simulink model "DSC_filtering"  (R2022a)
settings: Solver=FixedStepDiscrete  StartTime=0.0  StopTime=Inf  FixedStep=100e-6  RelTol=1e-3  EnableMultiTasking=on
undefined symbols (not defined in the file): Num
settings Model: ExtModeEnableFloating=off  ExtModeTrigType=signal  ExtModeTrigDuration=1001  ExtModeTrigLevel=0.500000  ExtModeArchiveMode=auto  ExtModeArchiveFileName=Simulation  ExtModeArchiveDirName=C:\Users\05983057\Documents\MATLAB\practica2\03_DSC  ExtModeLogAll=off  Creator=05983057  LastModifiedBy=05983057
settings DataIOCC: ReturnWorkspaceOutputs=off
settings OptimizationCC: DefaultUnderspecifiedDataType=single  EnhancedBackFolding=on  PassReuseOutputArgsAs=Individual arguments  MaxStackSize=1024  OptimizeBlockOrder=speed  DifferentSizesBufferReuse=on  OptimizationCustomize=off  DenormalBehavior=FlushToZero  EfficientTunableParamExpr=on
settings DebuggingCC: ParameterTunabilityLossMsg=error
settings HardwareCC: ProdBitPerChar=16  ProdBitPerInt=16  ProdBitPerPointer=32  ProdBitPerSizeT=32  ProdBitPerPtrDiffT=32  ProdLargestAtomicInteger=Integer  ProdLargestAtomicFloat=None  ProdWordSize=16  ProdLongLongMode=on  ProdHWDeviceType=Texas Instruments->C2000
settings SFSimCC: MATLABDynamicMemAlloc=off
settings RTWCC: SystemTargetFile=ert.tlc  HardwareBoard=TI Delfino F2833x  TemplateMakefile=ert_default_tmf  Toolchain=Texas Instruments Code Composer Studio (C2000)
settings CodeAppCC: ForceParamTrailComments=on  IgnoreCustomStorageClasses=off  OperatorAnnotations=on  SimulinkDataObjDesc=on  SFDataObjDesc=on  InsertBlockDesc=on
settings ERTTargetCC: CodeReplacementLibrary=TI C28x  ExtModeTransport=3

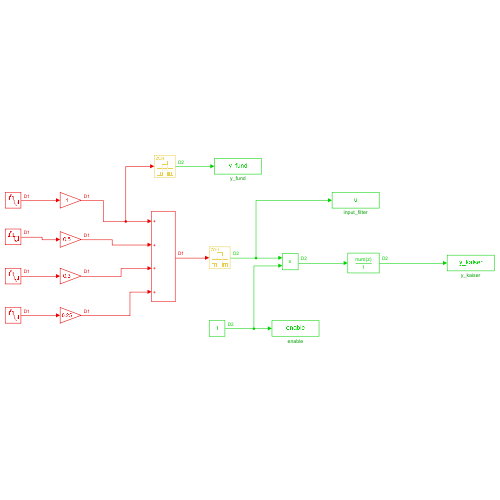
[thumbnail: Simulink's stored preview of the top-level diagram]
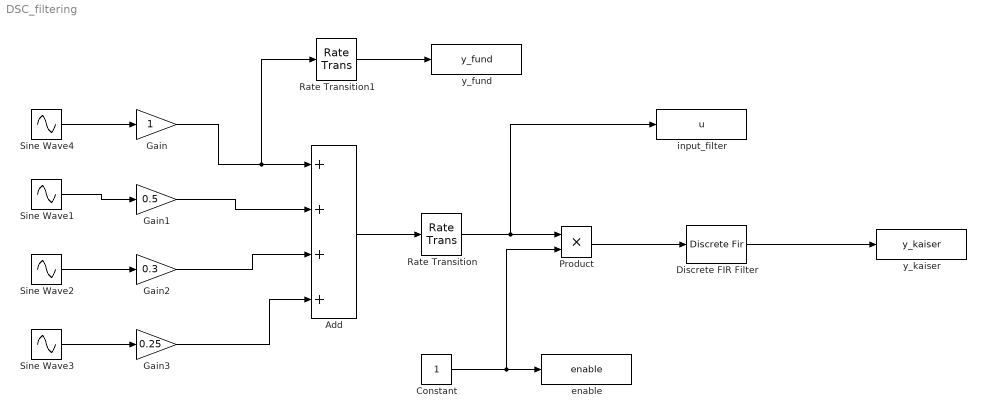
== system DSC_filtering ==
  Add : Sum  Inputs=4
  Constant : Constant  SampleTime=1/1e3
  Discrete FIR Filter : DiscreteFir  Coefficients=Num  SampleTime=1/1e3
  Gain : Gain
  Gain1 : Gain  Gain=0.5
  Gain2 : Gain  Gain=0.3
  Gain3 : Gain  Gain=0.25
  Product : Product
  Rate Transition : RateTransition  OutPortSampleTime=1e-3
  Rate Transition1 : RateTransition  OutPortSampleTime=1e-3
  Sine Wave1 : Sin  Frequency=150*2*pi  SampleTime=1/10e3
  Sine Wave2 : Sin  Frequency=250*2*pi  SampleTime=1/10e3
  Sine Wave3 : Sin  Frequency=350*2*pi  SampleTime=1/10e3
  Sine Wave4 : Sin  Frequency=50*2*pi  SampleTime=1/10e3
  enable : ToWorkspace  VariableName=enable  SampleTime=-1
  input_filter : ToWorkspace  VariableName=u  SampleTime=-1
  y_fund : ToWorkspace  VariableName=y_fund  SampleTime=-1
  y_kaiser : ToWorkspace  VariableName=y_kaiser  SampleTime=-1
  wires:
  Sine Wave4/1 -> Gain/1
  Sine Wave1/1 -> Gain1/1
  Sine Wave2/1 -> Gain2/1
  Sine Wave3/1 -> Gain3/1
  Gain/1 -> Rate Transition1/1, Add/1
  Gain1/1 -> Add/2
  Gain2/1 -> Add/3
  Gain3/1 -> Add/4
  Add/1 -> Rate Transition/1
  Constant/1 -> Product/2, enable/1
  Rate Transition/1 -> input_filter/1, Product/1
  Rate Transition1/1 -> y_fund/1
  Product/1 -> Discrete FIR Filter/1
  Discrete FIR Filter/1 -> y_kaiser/1
